simulink model "transformer_2"  (Simulink 7.4)
settings: Solver=ode45  StartTime=0.0  StopTime=1  RelTol=1e-3
libraries: powerlib x8, simulink x1
settings Model: Creator=dbenson  LastModifiedBy=dbenson

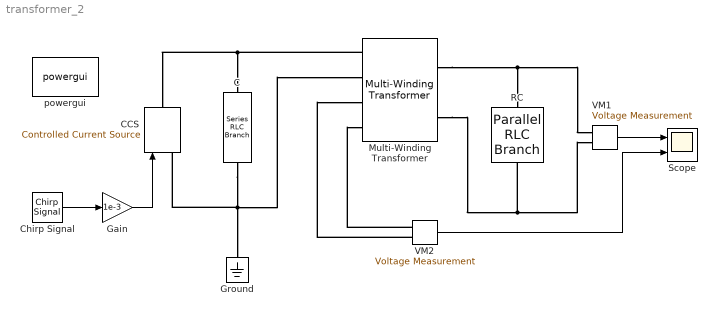
== system transformer_2 ==
  C : powerlib/Elements/Series RLC Branch  DialogController=POWERSYS.PowerSysDialog  PhysicalDomain=powersysdomain  SubClassName=unknown  LeftPortType=p1  RightPortType=p1  LConnTagsString=__new0  RConnTagsString=__new0  BranchType=C  Resistance=1  Inductance=1e-3  SetiL0=off  InitialCurrent=0  Capacitance=0.1e-6  Setx0=off  InitialVoltage=0  Measurements=None
  CCS : powerlib/Electrical Sources/Controlled Current Source  DialogController=POWERSYS.PowerSysDialog  SystemSampleTime=-1  Initialize=on  Source_Type=AC  Amplitude=0  Phase=0  Frequency=0  Measurements=None
  Chirp Signal : simulink/Sources/Chirp Signal  SystemSampleTime=-1  f1=10  T=10  f2=1000
  Gain : Gain  Gain=1e-3  ParameterDataType=fixdt(1, 16)  ParameterScaling=2^0  OutDataType=fixdt(1, 16)  OutScaling=2^0
  Ground : powerlib/Elements/Ground  DialogController=POWERSYS.PowerSysDialog  PhysicalDomain=powersysdomain  SubClassName=unknown  LeftPortType=p1  RightPortType=p1  LConnTagsString=a
  Multi-Winding Transformer : powerlib/Elements/Multi-Winding Transformer  DialogController=POWERSYS.PowerSysDialog  SystemSampleTime=-1  LeftWindings=2  RightWindings=1  TappedWindings=no taps  NumberOfTaps=2  UNITS=SI  NominalPower=[75e3 60]  NominalVoltages="[ 14400  120  120 120 ]"  WindingResistances=[13.824 0.00096 0.00096]  WindingInductances=[0.14668 1.0186e-005 1.0186e-005 1.0186e-005]  SetSaturation=off  Rm=1.3824e+005  Lm=366.69  Saturation=[0 0;0.017678 64.823;7.3657 82.109]  Hysteresis=off  DataFile='hysteresis.mat'  Measurements=None  MoreParameters=off  BreakLoop=off  DataType=on  InitialFlux=0  TransfoNumber=1
  RC : powerlib/Elements/Parallel RLC Branch  DialogController=POWERSYS.PowerSysDialog  PhysicalDomain=powersysdomain  SubClassName=unknown  LeftPortType=p1  RightPortType=p1  LConnTagsString=a  RConnTagsString=__new0  BranchType=RC  Resistance=1000  Inductance=1e-3  SetiL0=off  InitialCurrent=0  Capacitance=100e-9  Setx0=off  InitialVoltage=0  Measurements=None
  Scope : Scope  NumInputPorts=2
      settings: TimeRange=1  YMin=-2~-2  YMax=2~2  MaxDataPoints=500000
  VM1 : powerlib/Measurements/Voltage Measurement  DialogController=POWERSYS.PowerSysDialog  SystemSampleTime=-1  PhasorSimulation=off  OutputType=Complex  PSBequivalent=0
  VM2 : powerlib/Measurements/Voltage Measurement  DialogController=POWERSYS.PowerSysDialog  SystemSampleTime=-1  PhasorSimulation=off  OutputType=Complex  PSBequivalent=0
  powergui : powerlib/powergui  Priority=1  SystemSampleTime=-1  SimulationMode=Continuous  SampleTime=50e-6  frequency=60  SPID=off  DisableSnubberDevices=off  DisableRonSwitches=off  DisableVfSwitches=off  SwTol=0  Interpol=off  frequencyindice=0  echomessages=off  HookPort=off  DisplayEquations=off  FunctionMessages=off  EnableUseOfTLC=off  x0status=blocks  RestoreLinks=warning  Frange=[0:2:500]  Ylog=off  Xlog=on  ShowGrid=off  save=off  variable=ZData  ZoomFFT=on  StartTime=0.0  cycles=1  DisplayStyle=1  fundamental=60  FreqAxis=off  MaxFrequency=1000  frequencyindicesteady=1  RmsSteady=1  display=off  Ts=0  methode=off
  wires:
  Chirp Signal/1 -> Gain/1
  VM1/1 -> Scope/1
  VM2/1 -> Scope/2
  Gain/1 -> CCS/1
  connections:
  Multi-Winding Transformer/LConn1 -- CCS/RConn1 -- C/LConn1
  VM2/LConn2 -- Multi-Winding Transformer/LConn3
  VM2/LConn1 -- Multi-Winding Transformer/LConn4
  Multi-Winding Transformer/RConn1 -- RC/LConn1 -- VM1/LConn1
  Multi-Winding Transformer/RConn2 -- RC/RConn1 -- VM1/LConn2
  C/RConn1 -- Multi-Winding Transformer/LConn2 -- Ground/LConn1 -- CCS/LConn1
